simulink model "sistema"  (R2023a)
settings: Solver=VariableStepAuto  StartTime=0.0  StopTime=10.0  RelTol=1e-3
settings Model: Creator=Jose Venegas  LastModifiedBy=Jose Venegas
settings DataIOCC: SaveOutput=off  SignalLogging=off  DSMLogging=off  ReturnWorkspaceOutputs=off  TimeSaveName=t
settings DebuggingCC: AlgebraicLoopMsg=none  ArtificialAlgebraicLoopMsg=none  MaxConsecutiveZCsMsg=none  ModelReferenceExtraNoncontSigs=none  OperatingPointInterfaceChecksumMismatchMsg=none

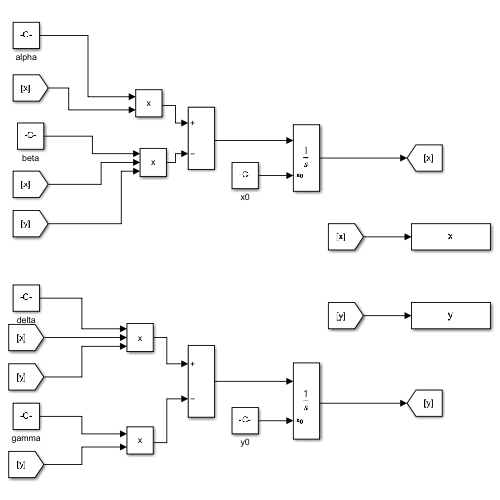
[thumbnail: Simulink's stored preview of the top-level diagram]
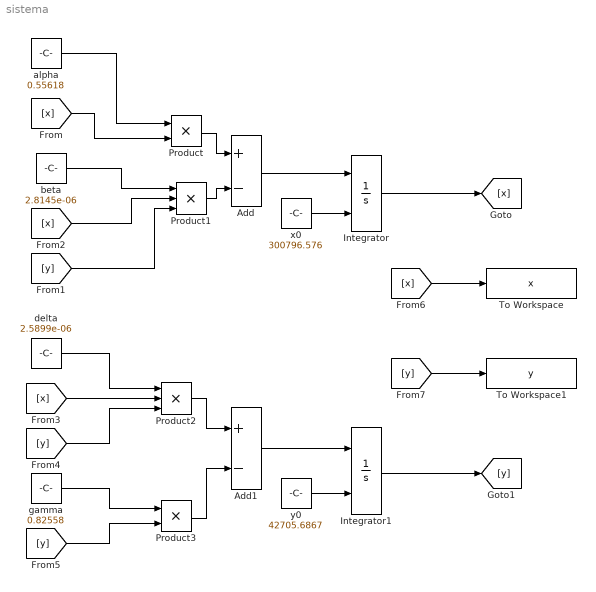
== system sistema ==
  Add : Sum  Inputs=+-
  Add1 : Sum  Inputs=+-
  Integrator : Integrator  InitialConditionSource=external
  Integrator1 : Integrator  InitialConditionSource=external
  Product : Product
  Product1 : Product  Inputs=3
  Product2 : Product  Inputs=3
  Product3 : Product
  To Workspace : ToWorkspace  VariableName=x  SampleTime=-1
  To Workspace1 : ToWorkspace  VariableName=y  SampleTime=-1
  alpha : Constant  Value=0.55618
  beta : Constant  Value=2.8145e-06
  delta : Constant  Value=2.5899e-06
  gamma : Constant  Value=0.82558
  x0 : Constant  Value=300796.576
  y0 : Constant  Value=42705.6867
  wires:
  x0/1 -> Integrator/2
  Add/1 -> Integrator/1
  Integrator/1 -> [x]
  Integrator1/1 -> [y]
  Add1/1 -> Integrator1/1
  y0/1 -> Integrator1/2
  alpha/1 -> Product/1
  [x] -> Product/2
  Product/1 -> Add/1
  beta/1 -> Product1/1
  [x] -> Product1/2
  [y] -> Product1/3
  delta/1 -> Product2/1
  Product1/1 -> Add/2
  [x] -> Product2/2
  [y] -> Product2/3
  [y] -> Product3/2
  gamma/1 -> Product3/1
  Product2/1 -> Add1/1
  Product3/1 -> Add1/2
  [x] -> To Workspace/1
  [y] -> To Workspace1/1
